simulink model "digital_com_2nd_lab"  (R2022b)
settings: Solver=VariableStepAuto  StartTime=0.0  StopTime=10.0  RelTol=1e-3
libraries: simulink x1, spsMonostableLib x1
settings Model: Creator=Asus  LastModifiedBy=Asus

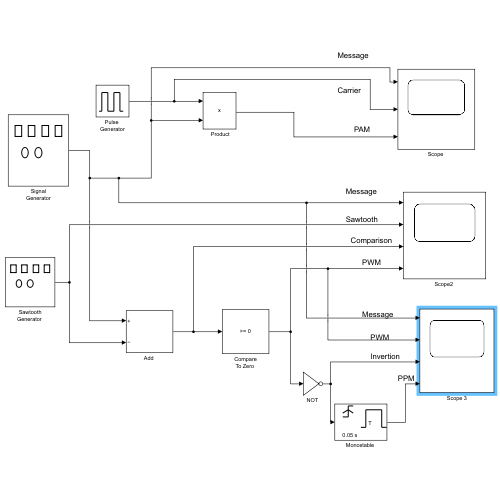
[thumbnail: Simulink's stored preview of the top-level diagram]
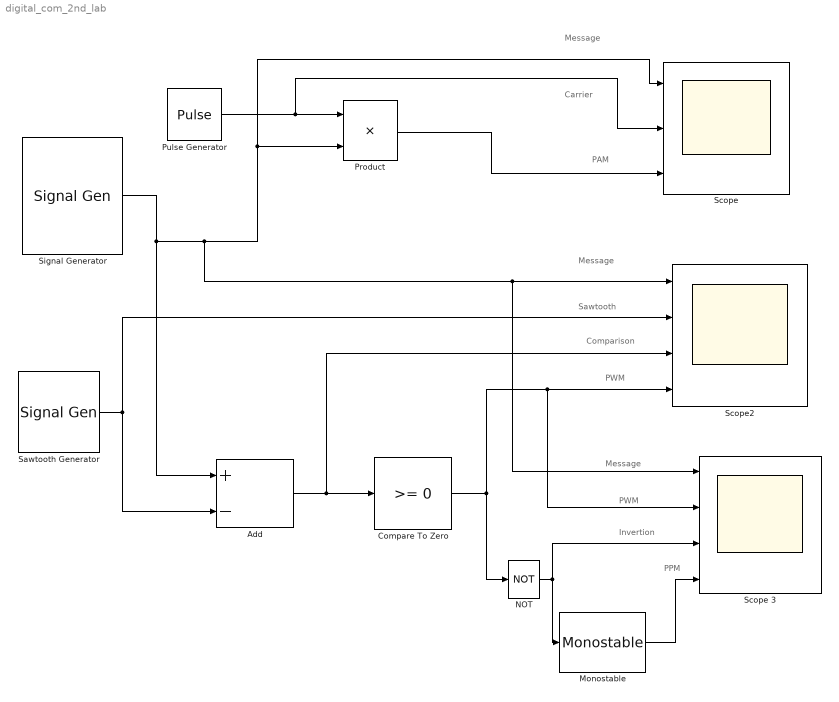
== system digital_com_2nd_lab ==
  note: Message
  note: Carrier
  note: PAM
  note: Message
  note: Sawtooth
  note: Comparison
  note: PWM
  note: PWM
  note: Message
  note: Invertion
  note: PPM
  " Product" : Product
  "Add " : Sum  Inputs=+-
  "Compare To Zero " : simulink/Logic and Bit Operations/Compare To Zero  relop=>=  OutDataTypeStr=boolean
  "Monostable " : spsMonostableLib/Monostable  EdgeDetect=Rising  PulseDuration=0.05  ic=0  Ts=0
      settings: LibrarySourceBlock=sps_lib/Control/Monostable
  "NOT " : Logic  Operator=NOT  IconShape=distinctive  AllPortsSameDT=off  OutDataTypeStr=boolean
  Pulse Generator : DiscretePulseGenerator  PulseType=Time based  Period=0.1  PulseWidth=5
  "Sawtooth Generator " : SignalGenerator  WaveForm=sawtooth  Frequency=5  Units=rad/sec
  "Scope " : Scope  NumInputPorts=3
  Scope 3 : Scope  NumInputPorts=4
  "Scope2 " : Scope  NumInputPorts=4
  Signal Generator : SignalGenerator  Amplitude=0.9  Units=rad/sec
  wires:
  Pulse Generator/1 -> "Scope "/2, " Product"/1
  Signal Generator/1 -> "Add "/1, Scope 3/1, "Scope2 "/1, "Scope "/1, " Product"/2
  " Product"/1 -> "Scope "/3
  "Sawtooth Generator "/1 -> "Add "/2, "Scope2 "/2
  "Add "/1 -> "Scope2 "/3, "Compare To Zero "/1
  "Compare To Zero "/1 -> "NOT "/1, Scope 3/2, "Scope2 "/4
  "NOT "/1 -> "Monostable "/1, Scope 3/3
  "Monostable "/1 -> Scope 3/4
